simulink model "untitled1"  (R2020a)
settings: Solver=VariableStepAuto  StartTime=0.0  StopTime=10.0  RelTol=1e-3
settings Model: Creator=isz8  LastModifiedBy=isz8

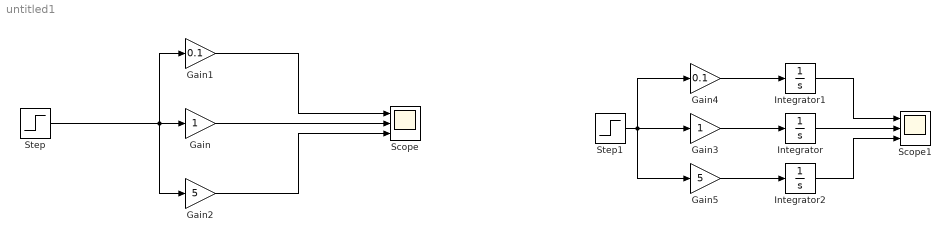
== system untitled1 ==
  Gain : Gain
  Gain1 : Gain  Gain=0.1
  Gain2 : Gain  Gain=5
  Gain3 : Gain
  Gain4 : Gain  Gain=0.1
  Gain5 : Gain  Gain=5
  Integrator : Integrator
  Integrator1 : Integrator
  Integrator2 : Integrator
  Scope : Scope  NumInputPorts=3
  Scope1 : Scope  NumInputPorts=3
  Step : Step  SampleTime=0
  Step1 : Step  SampleTime=0
  wires:
  Step/1 -> Gain2/1, Gain1/1, Gain/1
  Gain1/1 -> Scope/1
  Gain2/1 -> Scope/3
  Gain/1 -> Scope/2
  Step1/1 -> Gain5/1, Gain4/1, Gain3/1
  Gain3/1 -> Integrator/1
  Gain4/1 -> Integrator1/1
  Gain5/1 -> Integrator2/1
  Integrator1/1 -> Scope1/1
  Integrator/1 -> Scope1/2
  Integrator2/1 -> Scope1/3
